simulink model "acac_robust_optimized_r2024a"  (R2024a)
settings: Solver=daessc  StartTime=0  StopTime=0.4  MaxStep=1e-6  RelTol=1e-4
model workspace (MAT data in the model file):
  Fout_Hz = 30
libraries: fl_lib x40, nesl_utility x27, ee_lib x11
(part 1 of 2)
settings Model: Creator=chidan  LastModifiedBy=chidan

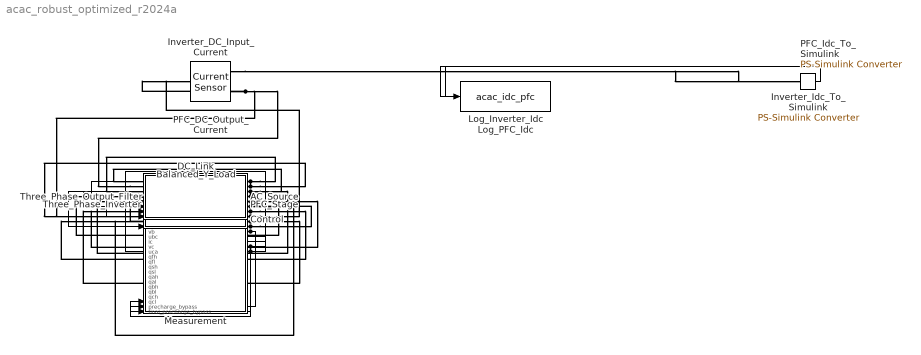
== system acac_robust_optimized_r2024a ==
  AC_Source : Subsystem
  Balanced_Y_Load : Subsystem
  Control : Subsystem
  DC_Link : Subsystem
  Inverter_DC_Input_Current : fl_lib/Electrical/Electrical Sensors/Current Sensor
  Inverter_Idc_To_Simulink : nesl_utility/PS-Simulink Converter  PhysicalDomain=network_engine_domain  SubClassName=ps_output  LeftPortType=input  RightPortType=output  PseudoPeriodic=off  Frequencies=[]  VectorFormat=inherit  Unit=A  AffineConversion=off
  Log_Inverter_Idc : ToWorkspace  VariableName=acac_idc_inverter  SaveFormat=Timeseries  SampleTime=-1
  Log_PFC_Idc : ToWorkspace  VariableName=acac_idc_pfc  SaveFormat=Timeseries  SampleTime=-1
  Measurement : Subsystem
  PFC_DC_Output_Current : fl_lib/Electrical/Electrical Sensors/Current Sensor
  PFC_Idc_To_Simulink : nesl_utility/PS-Simulink Converter  PhysicalDomain=network_engine_domain  SubClassName=ps_output  LeftPortType=input  RightPortType=output  PseudoPeriodic=off  Frequencies=[]  VectorFormat=inherit  Unit=A  AffineConversion=off
  PFC_Stage : Subsystem
  Three_Phase_Inverter : Subsystem
  Three_Phase_Output_Filter : Subsystem
  wires:
  Control/1(QFH) -> PFC_Stage/1(Gate_QFH), Measurement/15(qfh)
  Control/2(QFL) -> PFC_Stage/2(Gate_QFL), Measurement/16(qfl)
  Control/3(QSH) -> PFC_Stage/3(Gate_QSH), Measurement/17(qsh)
  Control/4(QSL) -> PFC_Stage/4(Gate_QSL), Measurement/18(qsl)
  Control/5(QAH) -> Three_Phase_Inverter/1(Gate_AH), Measurement/19(qah)
  Control/6(QAL) -> Three_Phase_Inverter/2(Gate_AL), Measurement/20(qal)
  Control/7(QBH) -> Three_Phase_Inverter/3(Gate_BH), Measurement/21(qbh)
  Control/8(QBL) -> Three_Phase_Inverter/4(Gate_BL), Measurement/22(qbl)
  Control/9(QCH) -> Three_Phase_Inverter/5(Gate_CH), Measurement/23(qch)
  Control/10(QCL) -> Three_Phase_Inverter/6(Gate_CL), Measurement/24(qcl)
  PFC_Stage/1(vin) -> Control/1(vin), Measurement/1(vin)
  PFC_Stage/2(iin) -> Control/2(iin), Measurement/2(iin)
  PFC_Stage/3(vdc) -> Control/3(vdc), Measurement/3(vdc)
  Balanced_Y_Load/2(Va) -> Control/4(va), Measurement/7(va)
  Control/11(PFC_Duty) -> Measurement/4(pfc_duty)
  Control/12(Inverter_Modulation) -> Measurement/5(inverter_modulation)
  Balanced_Y_Load/1(Ia) -> Measurement/6(ia)
  Balanced_Y_Load/3(Uab) -> Measurement/8(uab)
  Balanced_Y_Load/4(Ib) -> Measurement/9(ib)
  Balanced_Y_Load/5(Vb) -> Measurement/10(vb), Control/5(Sense_vb)
  Balanced_Y_Load/6(Ubc) -> Measurement/11(ubc)
  Balanced_Y_Load/7(Ic) -> Measurement/12(ic)
  Balanced_Y_Load/8(Vc) -> Measurement/13(vc), Control/6(Sense_vc)
  Balanced_Y_Load/9(Uca) -> Measurement/14(uca)
  Control/13(Precharge_Bypass) -> PFC_Stage/5(Gate_Precharge_Bypass), Measurement/25(precharge_bypass)
  Control/14(Final_Precharge_Bypass) -> PFC_Stage/6(Gate_Final_Precharge_Bypass), Measurement/26(final_precharge_bypass)
  Inverter_Idc_To_Simulink/1 -> Log_Inverter_Idc/1
  PFC_Idc_To_Simulink/1 -> Log_PFC_Idc/1
  connections:
  AC_Source/RConn1 -- PFC_Stage/LConn1
  AC_Source/RConn2 -- PFC_Stage/LConn2
  DC_Link/LConn2 -- PFC_Stage/RConn2 -- Three_Phase_Inverter/LConn2
  Three_Phase_Inverter/RConn1 -- Three_Phase_Output_Filter/LConn1
  Three_Phase_Inverter/RConn2 -- Three_Phase_Output_Filter/LConn2
  Three_Phase_Inverter/RConn3 -- Three_Phase_Output_Filter/LConn3
  Three_Phase_Output_Filter/RConn1 -- Balanced_Y_Load/LConn1
  Three_Phase_Output_Filter/RConn2 -- Balanced_Y_Load/LConn2
  Three_Phase_Output_Filter/RConn3 -- Balanced_Y_Load/LConn3
  Three_Phase_Output_Filter/RConn4 -- Balanced_Y_Load/LConn4
  Inverter_DC_Input_Current/RConn2 -- Three_Phase_Inverter/LConn1
  Inverter_DC_Input_Current/RConn1 -- Inverter_Idc_To_Simulink/LConn1
  PFC_Stage/RConn1 -- PFC_DC_Output_Current/LConn1
  DC_Link/LConn1 -- PFC_DC_Output_Current/RConn2 -- Inverter_DC_Input_Current/LConn1
  PFC_DC_Output_Current/RConn1 -- PFC_Idc_To_Simulink/LConn1

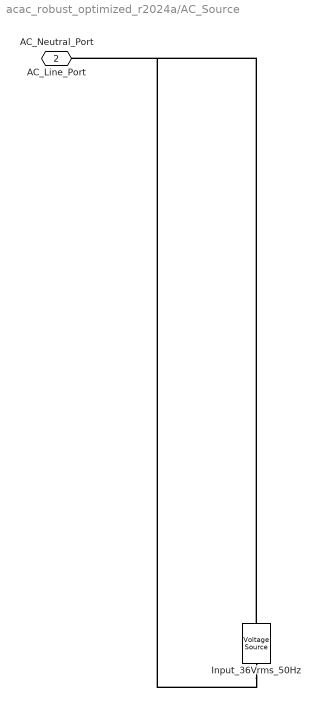
== system acac_robust_optimized_r2024a/AC_Source ==
  Input_36Vrms_50Hz : ee_lib/Sources/Voltage Source  dc_voltage=0 V  ac_voltage=36*sqrt(2) V  ac_shift=0 rad  ac_frequency=50 Hz  noise_mode=ee.enum.sources.noise.Disabled  PSD=0 V^2/Hz  sample_time=1e-3 s  repeatability=ee.enum.sources.repeatability.NotRepeatable  user_seed=0  auto_seed=3499211588  i_specify=off  i_priority=None  i=0 A  i_nominal_specify=off  i_nominal_value=1  i_nominal_unit=A  v_specify=off  v_priority=None  v=0 V  v_nominal_specify=off  v_nominal_value=1  v_nominal_unit=V
  AC_Line_Port : PMIOPort  Side=Right
  AC_Neutral_Port : PMIOPort  Port=2  Side=Right
  connections:
  Input_36Vrms_50Hz/LConn1 -- AC_Line_Port/RConn1
  Input_36Vrms_50Hz/RConn1 -- AC_Neutral_Port/RConn1

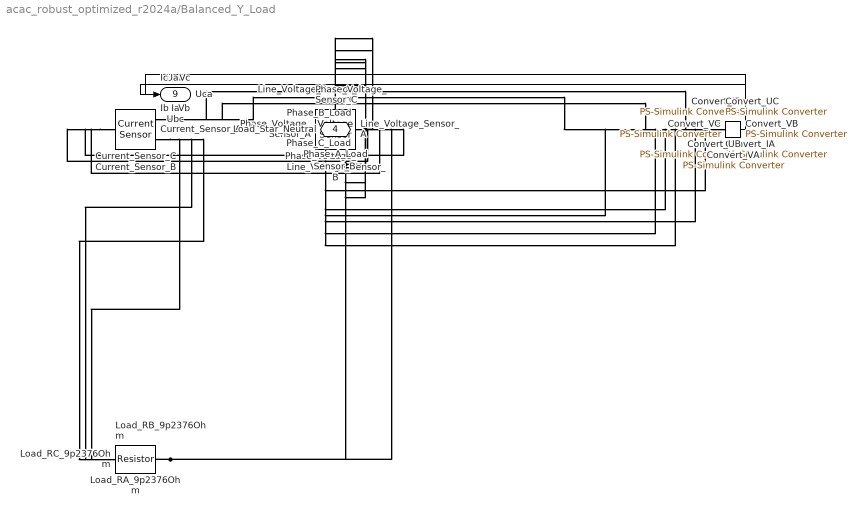
== system acac_robust_optimized_r2024a/Balanced_Y_Load ==
  Convert_IA : nesl_utility/PS-Simulink Converter  PhysicalDomain=network_engine_domain  SubClassName=ps_output  LeftPortType=input  RightPortType=output  PseudoPeriodic=off  Frequencies=[]  VectorFormat=inherit  Unit=inherit  AffineConversion=off
  Convert_IB : nesl_utility/PS-Simulink Converter  PhysicalDomain=network_engine_domain  SubClassName=ps_output  LeftPortType=input  RightPortType=output  PseudoPeriodic=off  Frequencies=[]  VectorFormat=inherit  Unit=inherit  AffineConversion=off
  Convert_IC : nesl_utility/PS-Simulink Converter  PhysicalDomain=network_engine_domain  SubClassName=ps_output  LeftPortType=input  RightPortType=output  PseudoPeriodic=off  Frequencies=[]  VectorFormat=inherit  Unit=inherit  AffineConversion=off
  Convert_UA : nesl_utility/PS-Simulink Converter  PhysicalDomain=network_engine_domain  SubClassName=ps_output  LeftPortType=input  RightPortType=output  PseudoPeriodic=off  Frequencies=[]  VectorFormat=inherit  Unit=inherit  AffineConversion=off
  Convert_UB : nesl_utility/PS-Simulink Converter  PhysicalDomain=network_engine_domain  SubClassName=ps_output  LeftPortType=input  RightPortType=output  PseudoPeriodic=off  Frequencies=[]  VectorFormat=inherit  Unit=inherit  AffineConversion=off
  Convert_UC : nesl_utility/PS-Simulink Converter  PhysicalDomain=network_engine_domain  SubClassName=ps_output  LeftPortType=input  RightPortType=output  PseudoPeriodic=off  Frequencies=[]  VectorFormat=inherit  Unit=inherit  AffineConversion=off
  Convert_VA : nesl_utility/PS-Simulink Converter  PhysicalDomain=network_engine_domain  SubClassName=ps_output  LeftPortType=input  RightPortType=output  PseudoPeriodic=off  Frequencies=[]  VectorFormat=inherit  Unit=inherit  AffineConversion=off
  Convert_VB : nesl_utility/PS-Simulink Converter  PhysicalDomain=network_engine_domain  SubClassName=ps_output  LeftPortType=input  RightPortType=output  PseudoPeriodic=off  Frequencies=[]  VectorFormat=inherit  Unit=inherit  AffineConversion=off
  Convert_VC : nesl_utility/PS-Simulink Converter  PhysicalDomain=network_engine_domain  SubClassName=ps_output  LeftPortType=input  RightPortType=output  PseudoPeriodic=off  Frequencies=[]  VectorFormat=inherit  Unit=inherit  AffineConversion=off
  Current_Sensor_A : fl_lib/Electrical/Electrical Sensors/Current Sensor
  Current_Sensor_B : fl_lib/Electrical/Electrical Sensors/Current Sensor
  Current_Sensor_C : fl_lib/Electrical/Electrical Sensors/Current Sensor
  Line_Voltage_Sensor_A : fl_lib/Electrical/Electrical Sensors/Voltage Sensor
  Line_Voltage_Sensor_B : fl_lib/Electrical/Electrical Sensors/Voltage Sensor
  Line_Voltage_Sensor_C : fl_lib/Electrical/Electrical Sensors/Voltage Sensor
  Load_RA_9p2376Ohm : fl_lib/Electrical/Electrical Elements/Resistor  R=9.237604307 Ohm  i_specify=off  i_priority=None  i=0 A  i_nominal_specify=off  i_nominal_value=1  i_nominal_unit=A  v_specify=off  v_priority=None  v=0 V  v_nominal_specify=off  v_nominal_value=1  v_nominal_unit=V
  Load_RB_9p2376Ohm : fl_lib/Electrical/Electrical Elements/Resistor  R=9.237604307 Ohm  i_specify=off  i_priority=None  i=0 A  i_nominal_specify=off  i_nominal_value=1  i_nominal_unit=A  v_specify=off  v_priority=None  v=0 V  v_nominal_specify=off  v_nominal_value=1  v_nominal_unit=V
  Load_RC_9p2376Ohm : fl_lib/Electrical/Electrical Elements/Resistor  R=9.237604307 Ohm  i_specify=off  i_priority=None  i=0 A  i_nominal_specify=off  i_nominal_value=1  i_nominal_unit=A  v_specify=off  v_priority=None  v=0 V  v_nominal_specify=off  v_nominal_value=1  v_nominal_unit=V
  Phase_Voltage_Sensor_A : fl_lib/Electrical/Electrical Sensors/Voltage Sensor
  Phase_Voltage_Sensor_B : fl_lib/Electrical/Electrical Sensors/Voltage Sensor
  Phase_Voltage_Sensor_C : fl_lib/Electrical/Electrical Sensors/Voltage Sensor
  Phase_A_Load : PMIOPort  Side=Left
  Phase_B_Load : PMIOPort  Port=2  Side=Left
  Phase_C_Load : PMIOPort  Port=3  Side=Left
  Load_Star_Neutral : PMIOPort  Port=4  Side=Left
  Ia : Outport
  Va : Outport  Port=2
  Uab : Outport  Port=3
  Ib : Outport  Port=4
  Vb : Outport  Port=5
  Ubc : Outport  Port=6
  Ic : Outport  Port=7
  Vc : Outport  Port=8
  Uca : Outport  Port=9
  wires:
  Convert_IA/1 -> Ia/1
  Convert_VA/1 -> Va/1
  Convert_IB/1 -> Ib/1
  Convert_VB/1 -> Vb/1
  Convert_IC/1 -> Ic/1
  Convert_VC/1 -> Vc/1
  Convert_UA/1 -> Uab/1
  Convert_UB/1 -> Ubc/1
  Convert_UC/1 -> Uca/1
  connections:
  Current_Sensor_A/LConn1 -- Phase_A_Load/RConn1 -- Phase_Voltage_Sensor_A/LConn1 -- Line_Voltage_Sensor_A/LConn1 -- Line_Voltage_Sensor_C/RConn2
  Current_Sensor_A/RConn2 -- Load_RA_9p2376Ohm/LConn1
  Phase_Voltage_Sensor_A/RConn2 -- Load_Star_Neutral/RConn1 -- Load_RA_9p2376Ohm/RConn1 -- Phase_Voltage_Sensor_B/RConn2 -- Phase_Voltage_Sensor_C/RConn2 -- Load_RB_9p2376Ohm/RConn1 -- Load_RC_9p2376Ohm/RConn1
  Current_Sensor_B/LConn1 -- Phase_B_Load/RConn1 -- Phase_Voltage_Sensor_B/LConn1 -- Line_Voltage_Sensor_A/RConn2 -- Line_Voltage_Sensor_B/LConn1
  Current_Sensor_B/RConn2 -- Load_RB_9p2376Ohm/LConn1
  Current_Sensor_C/LConn1 -- Phase_C_Load/RConn1 -- Phase_Voltage_Sensor_C/LConn1 -- Line_Voltage_Sensor_B/RConn2 -- Line_Voltage_Sensor_C/LConn1
  Current_Sensor_C/RConn2 -- Load_RC_9p2376Ohm/LConn1
  Current_Sensor_A/RConn1 -- Convert_IA/LConn1
  Current_Sensor_B/RConn1 -- Convert_IB/LConn1
  Current_Sensor_C/RConn1 -- Convert_IC/LConn1
  Phase_Voltage_Sensor_A/RConn1 -- Convert_VA/LConn1
  Phase_Voltage_Sensor_B/RConn1 -- Convert_VB/LConn1
  Phase_Voltage_Sensor_C/RConn1 -- Convert_VC/LConn1
  Line_Voltage_Sensor_A/RConn1 -- Convert_UA/LConn1
  Line_Voltage_Sensor_B/RConn1 -- Convert_UB/LConn1
  Line_Voltage_Sensor_C/RConn1 -- Convert_UC/LConn1

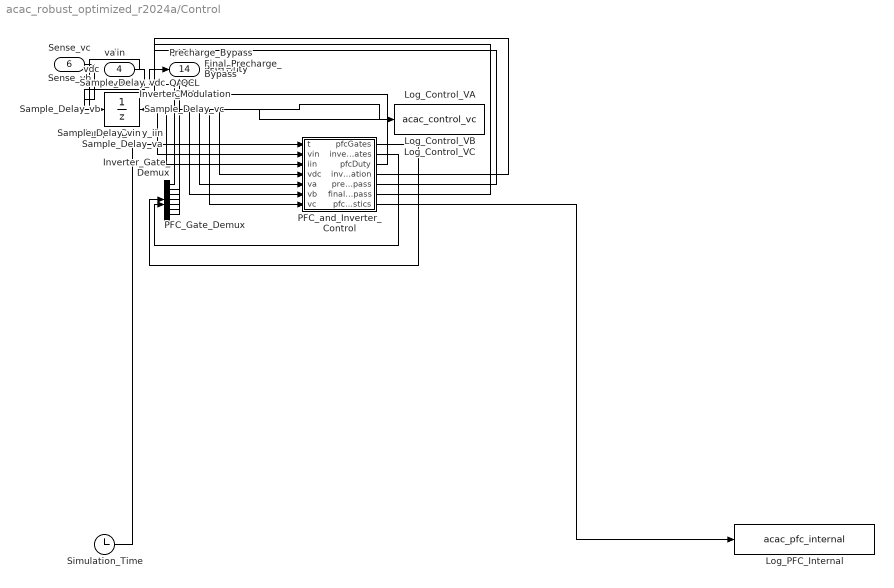
== system acac_robust_optimized_r2024a/Control ==
  vin : Inport
  iin : Inport  Port=2
  vdc : Inport  Port=3
  va : Inport  Port=4
  Sense_vb : Inport  Port=5
  Sense_vc : Inport  Port=6
  Inverter_Gate_Demux : Demux  Outputs=6
  Log_Control_VA : ToWorkspace  VariableName=acac_control_va  SaveFormat=Timeseries  SampleTime=-1
  Log_Control_VB : ToWorkspace  VariableName=acac_control_vb  SaveFormat=Timeseries  SampleTime=-1
  Log_Control_VC : ToWorkspace  VariableName=acac_control_vc  SaveFormat=Timeseries  SampleTime=-1
  Log_PFC_Internal : ToWorkspace  VariableName=acac_pfc_internal  SaveFormat=Timeseries  SampleTime=-1
      settings: Decimation=10
  PFC_Gate_Demux : Demux
  PFC_and_Inverter_Control : MATLAB Function  TreatAsAtomicUnit=on  SystemSampleTime=1e-6
  Sample_Delay_iin : UnitDelay  SampleTime=1e-6  HasFrameUpgradeWarning=on
  Sample_Delay_va : UnitDelay  SampleTime=1e-6  HasFrameUpgradeWarning=on
  Sample_Delay_vb : UnitDelay  SampleTime=1e-6  HasFrameUpgradeWarning=on
  Sample_Delay_vc : UnitDelay  SampleTime=1e-6  HasFrameUpgradeWarning=on
  Sample_Delay_vdc : UnitDelay  SampleTime=1e-6  HasFrameUpgradeWarning=on
  Sample_Delay_vin : UnitDelay  SampleTime=1e-6  HasFrameUpgradeWarning=on
  Simulation_Time : Clock
  QFH : Outport
  QFL : Outport  Port=2
  QSH : Outport  Port=3
  QSL : Outport  Port=4
  QAH : Outport  Port=5
  QAL : Outport  Port=6
  QBH : Outport  Port=7
  QBL : Outport  Port=8
  QCH : Outport  Port=9
  QCL : Outport  Port=10
  PFC_Duty : Outport  Port=11
  Inverter_Modulation : Outport  Port=12
  Precharge_Bypass : Outport  Port=13
  Final_Precharge_Bypass : Outport  Port=14
  wires:
  Simulation_Time/1 -> PFC_and_Inverter_Control/1(t)
  PFC_and_Inverter_Control/1(pfcGates) -> PFC_Gate_Demux/1
  PFC_and_Inverter_Control/2(inverterGates) -> Inverter_Gate_Demux/1
  PFC_and_Inverter_Control/3(pfcDuty) -> PFC_Duty/1
  PFC_and_Inverter_Control/4(inverterModulation) -> Inverter_Modulation/1
  PFC_Gate_Demux/1 -> QFH/1
  PFC_Gate_Demux/2 -> QFL/1
  PFC_Gate_Demux/3 -> QSH/1
  PFC_Gate_Demux/4 -> QSL/1
  Inverter_Gate_Demux/1 -> QAH/1
  Inverter_Gate_Demux/2 -> QAL/1
  Inverter_Gate_Demux/3 -> QBH/1
  Inverter_Gate_Demux/4 -> QBL/1
  Inverter_Gate_Demux/5 -> QCH/1
  Inverter_Gate_Demux/6 -> QCL/1
  vin/1 -> Sample_Delay_vin/1
  Sample_Delay_vin/1 -> PFC_and_Inverter_Control/2(vin)
  iin/1 -> Sample_Delay_iin/1
  Sample_Delay_iin/1 -> PFC_and_Inverter_Control/3(iin)
  vdc/1 -> Sample_Delay_vdc/1
  Sample_Delay_vdc/1 -> PFC_and_Inverter_Control/4(vdc)
  va/1 -> Sample_Delay_va/1
  Sample_Delay_va/1 -> PFC_and_Inverter_Control/5(va), Log_Control_VA/1
  PFC_and_Inverter_Control/5(prechargeBypass) -> Precharge_Bypass/1
  PFC_and_Inverter_Control/6(finalPrechargeBypass) -> Final_Precharge_Bypass/1
  Sense_vb/1 -> Sample_Delay_vb/1
  Sample_Delay_vb/1 -> PFC_and_Inverter_Control/6(vb), Log_Control_VB/1
  Sense_vc/1 -> Sample_Delay_vc/1
  Sample_Delay_vc/1 -> PFC_and_Inverter_Control/7(vc), Log_Control_VC/1
  PFC_and_Inverter_Control/7(pfcDiagnostics) -> Log_PFC_Internal/1

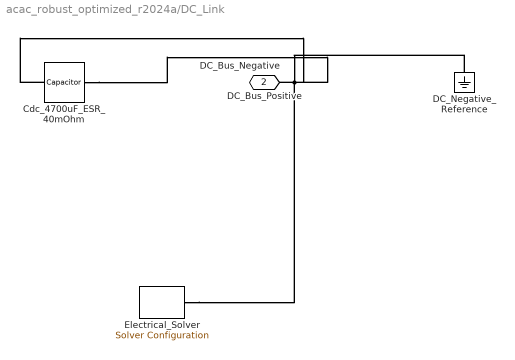
== system acac_robust_optimized_r2024a/DC_Link ==
  Cdc_4700uF_ESR_40mOhm : fl_lib/Electrical/Electrical Elements/Capacitor  c=4.7e-3 F  r=0.04 Ohm  g=0 1/Ohm  i_specify=off  i_priority=None  i=0 A  i_nominal_specify=off  i_nominal_value=1  i_nominal_unit=A  v_specify=off  v_priority=None  v=0 V  v_nominal_specify=off  v_nominal_value=1  v_nominal_unit=V  vc_specify=off  vc_priority=High  vc=0 V  vc_nominal_specify=off  vc_nominal_value=1  vc_nominal_unit=V
  DC_Negative_Reference : fl_lib/Electrical/Electrical Elements/Electrical Reference
  Electrical_Solver : nesl_utility/Solver Configuration  PhysicalDomain=network_engine_domain  SubClassName=solver  LeftPortType=input  RightPortType=generic  Tones=[]  Harmonics=[]  SimulateNoise=off  Profile=off  UseLocalSampling=off  EnableSwitchedLinearOptims=on  FrequencyDomain=off  UseCCode=off  RelTol=0.001  AbsTol=0.001  MinStep=1e-09  ToWorkspace=off  RevertToSquareIcSolve=off  NumHomotopyIterations=100  PhasorMode=off  PhasorModeNumHarmonics=1  ConsistencySolver=NEWTON_XTOL_AFTER_FTOL  IndexReductionMethod=DerivativeReplacement  DoDC=off  ResidualTolerance=1e-09  ConsistencyTolSource=GLOBAL  ConsistencyAbsTol=0.001  ConsistencyRelTol=0.001  ConsistencyTolFactor=0.001  UseLocalSolver=off  LocalSolverChoice=NE_BACKWARD_EULER_ADVANCER  ResolveIndetEquations=on  FunctionEvalNumThread=1  LocalSolverSampleTime=0.001  DoFixedCost=off  MaxNonlinIter=3  MaxModeIter=2  ComputeImpulses=off  ImpulseIterations=2  LinearAlgebra=auto  LinearAlgebraNumThread=0  EquationFormulation=NE_TIME_EF  DelaysMemoryBudget=1024  AutomaticFiltering=on  FilteringTimeConstant=0.001  PartitionStorageMethod=AS_NEEDED  PartitionMemoryBudget=1024  PartitionMethod=ROBUST  MultibodyUseLocalSolver=off  MultibodyLocalSolverChoice=ODE1  MultibodyLocalSolverSampleTime=0.001
  DC_Bus_Positive : PMIOPort  Side=Left
  DC_Bus_Negative : PMIOPort  Port=2  Side=Left
  connections:
  Cdc_4700uF_ESR_40mOhm/LConn1 -- DC_Bus_Positive/RConn1
  Cdc_4700uF_ESR_40mOhm/RConn1 -- DC_Negative_Reference/LConn1 -- DC_Bus_Negative/RConn1 -- Electrical_Solver/RConn1

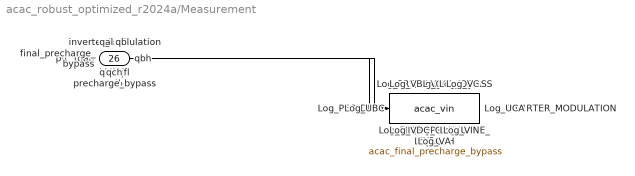
== system acac_robust_optimized_r2024a/Measurement ==
  vin : Inport
  iin : Inport  Port=2
  vdc : Inport  Port=3
  pfc_duty : Inport  Port=4
  inverter_modulation : Inport  Port=5
  ia : Inport  Port=6
  va : Inport  Port=7
  uab : Inport  Port=8
  ib : Inport  Port=9
  vb : Inport  Port=10
  ubc : Inport  Port=11
  ic : Inport  Port=12
  vc : Inport  Port=13
  uca : Inport  Port=14
  qfh : Inport  Port=15
  qfl : Inport  Port=16
  qsh : Inport  Port=17
  qsl : Inport  Port=18
  qah : Inport  Port=19
  qal : Inport  Port=20
  qbh : Inport  Port=21
  qbl : Inport  Port=22
  qch : Inport  Port=23
  qcl : Inport  Port=24
  precharge_bypass : Inport  Port=25
  final_precharge_bypass : Inport  Port=26
  Log_FINAL_PRECHARGE_BYPASS : ToWorkspace  VariableName=acac_final_precharge_bypass  SaveFormat=Timeseries  SampleTime=-1
  Log_IA : ToWorkspace  VariableName=acac_ia  SaveFormat=Timeseries  SampleTime=-1
  Log_IB : ToWorkspace  VariableName=acac_ib  SaveFormat=Timeseries  SampleTime=-1
  Log_IC : ToWorkspace  VariableName=acac_ic  SaveFormat=Timeseries  SampleTime=-1
  Log_IIN : ToWorkspace  VariableName=acac_iin  SaveFormat=Timeseries  SampleTime=-1
  Log_INVERTER_MODULATION : ToWorkspace  VariableName=acac_inverter_modulation  SaveFormat=Timeseries  SampleTime=-1
  Log_PFC_DUTY : ToWorkspace  VariableName=acac_pfc_duty  SaveFormat=Timeseries  SampleTime=-1
  Log_PRECHARGE_BYPASS : ToWorkspace  VariableName=acac_precharge_bypass  SaveFormat=Timeseries  SampleTime=-1
  Log_QAH : ToWorkspace  VariableName=acac_qah  SaveFormat=Timeseries  SampleTime=-1
  Log_QAL : ToWorkspace  VariableName=acac_qal  SaveFormat=Timeseries  SampleTime=-1
  Log_QBH : ToWorkspace  VariableName=acac_qbh  SaveFormat=Timeseries  SampleTime=-1
  Log_QBL : ToWorkspace  VariableName=acac_qbl  SaveFormat=Timeseries  SampleTime=-1
  Log_QCH : ToWorkspace  VariableName=acac_qch  SaveFormat=Timeseries  SampleTime=-1
  Log_QCL : ToWorkspace  VariableName=acac_qcl  SaveFormat=Timeseries  SampleTime=-1
  Log_QFH : ToWorkspace  VariableName=acac_qfh  SaveFormat=Timeseries  SampleTime=-1
  Log_QFL : ToWorkspace  VariableName=acac_qfl  SaveFormat=Timeseries  SampleTime=-1
  Log_QSH : ToWorkspace  VariableName=acac_qsh  SaveFormat=Timeseries  SampleTime=-1
  Log_QSL : ToWorkspace  VariableName=acac_qsl  SaveFormat=Timeseries  SampleTime=-1
  Log_UAB : ToWorkspace  VariableName=acac_uab  SaveFormat=Timeseries  SampleTime=-1
  Log_UBC : ToWorkspace  VariableName=acac_ubc  SaveFormat=Timeseries  SampleTime=-1
  Log_UCA : ToWorkspace  VariableName=acac_uca  SaveFormat=Timeseries  SampleTime=-1
  Log_VA : ToWorkspace  VariableName=acac_va  SaveFormat=Timeseries  SampleTime=-1
  Log_VB : ToWorkspace  VariableName=acac_vb  SaveFormat=Timeseries  SampleTime=-1
  Log_VC : ToWorkspace  VariableName=acac_vc  SaveFormat=Timeseries  SampleTime=-1
  Log_VDC : ToWorkspace  VariableName=acac_vdc  SaveFormat=Timeseries  SampleTime=-1
  Log_VIN : ToWorkspace  VariableName=acac_vin  SaveFormat=Timeseries  SampleTime=-1
  wires:
  vin/1 -> Log_VIN/1
  iin/1 -> Log_IIN/1
  vdc/1 -> Log_VDC/1
  pfc_duty/1 -> Log_PFC_DUTY/1
  inverter_modulation/1 -> Log_INVERTER_MODULATION/1
  ia/1 -> Log_IA/1
  va/1 -> Log_VA/1
  uab/1 -> Log_UAB/1
  ib/1 -> Log_IB/1
  vb/1 -> Log_VB/1
  ubc/1 -> Log_UBC/1
  ic/1 -> Log_IC/1
  vc/1 -> Log_VC/1
  uca/1 -> Log_UCA/1
  qfh/1 -> Log_QFH/1
  qfl/1 -> Log_QFL/1
  qsh/1 -> Log_QSH/1
  qsl/1 -> Log_QSL/1
  qah/1 -> Log_QAH/1
  qal/1 -> Log_QAL/1
  qbh/1 -> Log_QBH/1
  qbl/1 -> Log_QBL/1
  qch/1 -> Log_QCH/1
  qcl/1 -> Log_QCL/1
  precharge_bypass/1 -> Log_PRECHARGE_BYPASS/1
  final_precharge_bypass/1 -> Log_FINAL_PRECHARGE_BYPASS/1

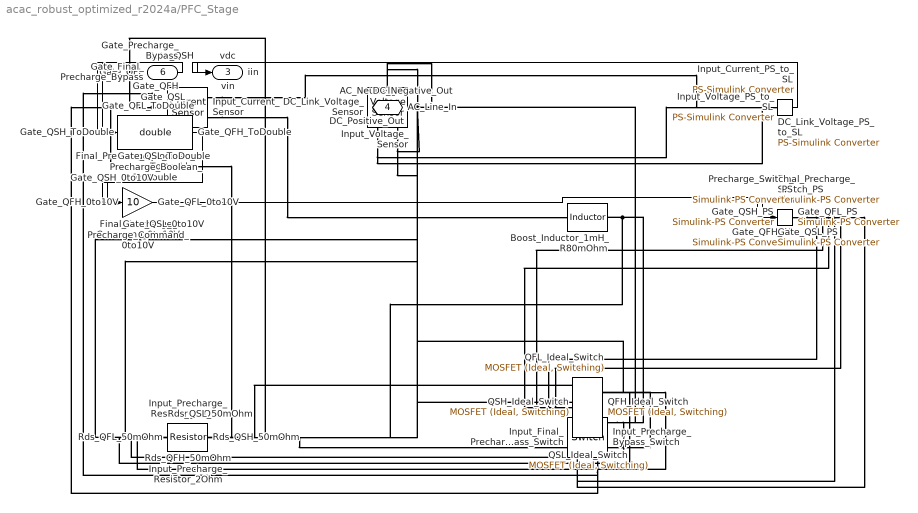
== system acac_robust_optimized_r2024a/PFC_Stage ==
  Gate_QFH : Inport
  Gate_QFL : Inport  Port=2
  Gate_QSH : Inport  Port=3
  Gate_QSL : Inport  Port=4
  Gate_Precharge_Bypass : Inport  Port=5
  Gate_Final_Precharge_Bypass : Inport  Port=6
  Boost_Inductor_1mH_R80mOhm : fl_lib/Electrical/Electrical Elements/Inductor  l=1e-3 H  r=0.08 Ohm  g=1e-9 1/Ohm  i_specify=off  i_priority=None  i=0 A  i_nominal_specify=off  i_nominal_value=1  i_nominal_unit=A  v_specify=off  v_priority=None  v=0 V  v_nominal_specify=off  v_nominal_value=1  v_nominal_unit=V  i_L_specify=off  i_L_priority=High  i_L=0 A  i_L_nominal_specify=off  i_L_nominal_value=1  i_L_nominal_unit=A
  DC_Link_Voltage_PS_to_SL : nesl_utility/PS-Simulink Converter  PhysicalDomain=network_engine_domain  SubClassName=ps_output  LeftPortType=input  RightPortType=output  PseudoPeriodic=off  Frequencies=[]  VectorFormat=inherit  Unit=inherit  AffineConversion=off
  DC_Link_Voltage_Sensor : fl_lib/Electrical/Electrical Sensors/Voltage Sensor
  Final_Precharge_Boolean_ToDouble : DataTypeConversion  OutDataTypeStr=double  SaturateOnIntegerOverflow=off  RndMeth=Floor
  Final_Precharge_Command_0to10V : Gain  Gain=10
  Final_Precharge_Switch_PS : nesl_utility/Simulink-PS Converter  PhysicalDomain=network_engine_domain  SubClassName=ps_input  LeftPortType=input  RightPortType=output  PseudoPeriodic=off  Frequencies=[]  NoiseDistribution=none  NoiseParameters=[]  Unit=1  AffineConversion=off  FilteringAndDerivatives=provide  SimscapeFilterOrder=1  InputFilterTimeConstant=0.001  UdotUserProvided=0
  Gate_QFH_0to10V : Gain  Gain=10
  Gate_QFH_PS : nesl_utility/Simulink-PS Converter  PhysicalDomain=network_engine_domain  SubClassName=ps_input  LeftPortType=input  RightPortType=output  PseudoPeriodic=off  Frequencies=[]  NoiseDistribution=none  NoiseParameters=[]  Unit=1  AffineConversion=off  FilteringAndDerivatives=provide  SimscapeFilterOrder=1  InputFilterTimeConstant=0.001  UdotUserProvided=0
  Gate_QFH_ToDouble : DataTypeConversion  OutDataTypeStr=double  SaturateOnIntegerOverflow=off  RndMeth=Floor
  Gate_QFL_0to10V : Gain  Gain=10
  Gate_QFL_PS : nesl_utility/Simulink-PS Converter  PhysicalDomain=network_engine_domain  SubClassName=ps_input  LeftPortType=input  RightPortType=output  PseudoPeriodic=off  Frequencies=[]  NoiseDistribution=none  NoiseParameters=[]  Unit=1  AffineConversion=off  FilteringAndDerivatives=provide  SimscapeFilterOrder=1  InputFilterTimeConstant=0.001  UdotUserProvided=0
  Gate_QFL_ToDouble : DataTypeConversion  OutDataTypeStr=double  SaturateOnIntegerOverflow=off  RndMeth=Floor
  Gate_QSH_0to10V : Gain  Gain=10
  Gate_QSH_PS : nesl_utility/Simulink-PS Converter  PhysicalDomain=network_engine_domain  SubClassName=ps_input  LeftPortType=input  RightPortType=output  PseudoPeriodic=off  Frequencies=[]  NoiseDistribution=none  NoiseParameters=[]  Unit=1  AffineConversion=off  FilteringAndDerivatives=provide  SimscapeFilterOrder=1  InputFilterTimeConstant=0.001  UdotUserProvided=0
  Gate_QSH_ToDouble : DataTypeConversion  OutDataTypeStr=double  SaturateOnIntegerOverflow=off  RndMeth=Floor
  Gate_QSL_0to10V : Gain  Gain=10
  Gate_QSL_PS : nesl_utility/Simulink-PS Converter  PhysicalDomain=network_engine_domain  SubClassName=ps_input  LeftPortType=input  RightPortType=output  PseudoPeriodic=off  Frequencies=[]  NoiseDistribution=none  NoiseParameters=[]  Unit=1  AffineConversion=off  FilteringAndDerivatives=provide  SimscapeFilterOrder=1  InputFilterTimeConstant=0.001  UdotUserProvided=0
  Gate_QSL_ToDouble : DataTypeConversion  OutDataTypeStr=double  SaturateOnIntegerOverflow=off  RndMeth=Floor
  Input_Current_PS_to_SL : nesl_utility/PS-Simulink Converter  PhysicalDomain=network_engine_domain  SubClassName=ps_output  LeftPortType=input  RightPortType=output  PseudoPeriodic=off  Frequencies=[]  VectorFormat=inherit  Unit=inherit  AffineConversion=off
  Input_Current_Sensor : fl_lib/Electrical/Electrical Sensors/Current Sensor
  Input_Final_Precharge_Bypass_Switch : fl_lib/Electrical/Electrical Elements/Switch  R_closed=0.01 Ohm  G_open=1e-8 1/Ohm  Threshold=0.5  i_specify=off  i_priority=None  i=0 A  i_nominal_specify=off  i_nominal_value=1  i_nominal_unit=A  v_specify=off  v_priority=None  v=0 V  v_nominal_specify=off  v_nominal_value=1  v_nominal_unit=V
  Input_Precharge_Bypass_Switch : fl_lib/Electrical/Electrical Elements/Switch  R_closed=0.01 Ohm  G_open=1e-8 1/Ohm  Threshold=0.5  i_specify=off  i_priority=None  i=0 A  i_nominal_specify=off  i_nominal_value=1  i_nominal_unit=A  v_specify=off  v_priority=None  v=0 V  v_nominal_specify=off  v_nominal_value=1  v_nominal_unit=V
  Input_Precharge_Resistor_10Ohm : fl_lib/Electrical/Electrical Elements/Resistor  R=10 Ohm  i_specify=off  i_priority=None  i=0 A  i_nominal_specify=off  i_nominal_value=1  i_nominal_unit=A  v_specify=off  v_priority=None  v=0 V  v_nominal_specify=off  v_nominal_value=1  v_nominal_unit=V
  Input_Precharge_Resistor_2Ohm : fl_lib/Electrical/Electrical Elements/Resistor  R=2 Ohm  i_specify=off  i_priority=None  i=0 A  i_nominal_specify=off  i_nominal_value=1  i_nominal_unit=A  v_specify=off  v_priority=None  v=0 V  v_nominal_specify=off  v_nominal_value=1  v_nominal_unit=V
  Input_Voltage_PS_to_SL : nesl_utility/PS-Simulink Converter  PhysicalDomain=network_engine_domain  SubClassName=ps_output  LeftPortType=input  RightPortType=output  PseudoPeriodic=off  Frequencies=[]  VectorFormat=inherit  Unit=inherit  AffineConversion=off
  Input_Voltage_Sensor : fl_lib/Electrical/Electrical Sensors/Voltage Sensor
  Precharge_Boolean_ToDouble : DataTypeConversion  OutDataTypeStr=double  SaturateOnIntegerOverflow=off  RndMeth=Floor
  Precharge_Command_0to10V : Gain  Gain=10
  Precharge_Switch_PS : nesl_utility/Simulink-PS Converter  PhysicalDomain=network_engine_domain  SubClassName=ps_input  LeftPortType=input  RightPortType=output  PseudoPeriodic=off  Frequencies=[]  NoiseDistribution=none  NoiseParameters=[]  Unit=1  AffineConversion=off  FilteringAndDerivatives=provide  SimscapeFilterOrder=1  InputFilterTimeConstant=0.001  UdotUserProvided=0
  QFH_Ideal_Switch : ee_lib/Semiconductors & Converters/MOSFET (Ideal, Switching)  port_option=ee.enum.controlport.ps  Rds=0.01 Ohm  Goff=1e-6 1/Ohm  Vth=2 V  diode_param=ee.enum.semiconductors.protectionDiode.nodynamics  diode_Vf=0.8 V  diode_Ron=0.001 Ohm  diode_Goff=1e-5 1/Ohm  diode_C=50e-9 F  diode_iRM=-235 A  diode_iF=300 A  diode_idot=-50 A/us  diode_trr_param=ee.enum.converters.diodeReverseParam.trr_factor  diode_trr_factor=3  diode_trr=15 us  diode_Qrr=1500 s*uA  ids_specify=off  ids_priority=None  ids=0 A  ids_nominal_specify=off  ids_nominal_value=1  ids_nominal_unit=A  vds_specify=off  vds_priority=None  vds=0 V  vds_nominal_specify=off  vds_nominal_value=1  vds_nominal_unit=V  vgs_specify=off  vgs_priority=None  vgs=0 V  vgs_nominal_specify=off  vgs_nominal_value=1  vgs_nominal_unit=V  thermal_loss_option=ee.enum.converters.thermalLossOption.constantvalues  Von_data=[0, 1.8, 3.2, 6, 10, 16; 0, 2, 5.5, 9.5, 15, 25] V  Tj=[298.15, 448.15] K  Iout_data=[0, 20, 40, 60, 80, 100] A  Eon_data=[0, 55.04, 124.57, 235.53, 362.12; 0, 71.25, 161.25, 304.88, 468.75] * 1e-6 J  Eoff_data=[0, 18, 30, 56.1, 76.5; 0, 22.5, 37.5, 70.13, 95.63] * 1e-6 J  Eon_data_3D=[zeros(2, 5, 3)] J  Eoff_data_3D=[zeros(2, 5, 3)] J  Tj_loss=[298.15, 448.15] K  Iout_data_loss=[0, 10, 20, 30, 40] A  tabulateWithVds=false  Vds_loss=[0, 150, 300] V  Eon_scalar=22.86e-3 J  Eoff_scalar=17.14e-3 J  Voff=300 V  Iout_scalar=600 A  useCurrentFromPreviousCycle=false  useVoltageFromPreviousCycle=false  diodeModelType=ee.enum.converters.diodeModelType.pwl  diodeTableType=ee.enum.diode.tableType.IfMat  diode_ReverseIVType=ee.enum.diode.diodeReverseIV.constant  diode_IfMat=[.07, .12, .19, 1.75, 4.24, 7.32, 11.2; .16, .3, .72, 2.14, 4.02, 6.35, 9.12] A  diode_VfMat=[.9, 1.15, 1.25, 1.5, 1.75, 2.17, 2.6, 2.85; .58, .68, .75, 1.1, 1.38, 1.77, 2.27, 2.7] V  diode_TjVec=[25, 125] degC  diode_VfVec=[.5, .7, .9, 1.3, 1.7, 2.1, 2.5] V  diode_IfVec=[.1, .2, .5, 1, 2, 4, 7, 10] A  diode_IrMat=[1e-06, 2e-06, 5e-06, 1e-05, 2.5e-05, 5e-05, .0001; 2e-06, 5e-06, 1e-05, 4e-05, 8e-05, .0002, .0005] A  diode_VrMat=[10, 100, 200, 250, 300, 325, 350; 10, 70, 160, 220, 270, 300, 320] V  diode_VrVec=[10, 20, 40, 50, 70, 80, 100] V  diode_IrVec=[1e-06, 2e-06, 5e-06, 1e-05, 2e-05, 5e-05, .0001] A  diode_Vr=-600 V  diode_Ls=150 nH  diode_Erec=0.03 J  diode_rec_loss_model=ee.enum.diode.reverseRecoveryModel.fixed  diode_ErecVal=0 J  diode_scaleWithIandV=true  diode_ErecMat=zeros(2, 3) J  diode_TjrecVec=[298.15, 398.15] K  diode_IfrecVec=[.1, 1, 10] A  diode_IrecVal=10 A  diode_VrecVal=10 V  diode_tFilter=1 / 1000 / 100 s  thermal_network_parameterization=ee.enum.thermalNetworkTopology.external  Rth=[.03, .2] K/W  Rth_Cauer=[.03, .1, .2] K/W  Rth_Foster=[.03, .2] K/W  thermal_mass_parameterization=ee.enum.thermalNetwork.timeconstant  thermal_mass=[3, 25] J/K  thermal_mass_Cauer=[3, 10, 25] J/K  thermal_mass_Foster=[33, 50] J/K  thermal_time_constant=[.1, 5] s  thermal_time_constant_Cauer=[.1, 1, 5] s  thermal_time_constant_Foster=[1, 10] s  thermal_mass_initial_temperatures=[25, 25] degC  thermal_mass_initial_temperatures_Cauer=[25, 25, 25] degC  junction_thermal_mass=0.1 J/K  Tvec_initial_Foster=[25, 25, 25, 25] degC  no_thermal_network=0  junction_temperature_specify=off  junction_temperature_priority=None  junction_temperature=25 degC  junction_temperature_nominal_specify=off  junction_temperature_nominal_value=1  junction_temperature_nominal_unit=degC  Qj_specify=off  Qj_priority=None  Qj=0 W  Qj_nominal_specify=off  Qj_nominal_value=1  Qj_nominal_unit=W  accumulatedSwitchingLosses_specify=off  accumulatedSwitchingLosses_priority=None  accumulatedSwitchingLosses=0 J
  QFL_Ideal_Switch : ee_lib/Semiconductors & Converters/MOSFET (Ideal, Switching)  port_option=ee.enum.controlport.ps  Rds=0.01 Ohm  Goff=1e-6 1/Ohm  Vth=2 V  diode_param=ee.enum.semiconductors.protectionDiode.nodynamics  diode_Vf=0.8 V  diode_Ron=0.001 Ohm  diode_Goff=1e-5 1/Ohm  diode_C=50e-9 F  diode_iRM=-235 A  diode_iF=300 A  diode_idot=-50 A/us  diode_trr_param=ee.enum.converters.diodeReverseParam.trr_factor  diode_trr_factor=3  diode_trr=15 us  diode_Qrr=1500 s*uA  ids_specify=off  ids_priority=None  ids=0 A  ids_nominal_specify=off  ids_nominal_value=1  ids_nominal_unit=A  vds_specify=off  vds_priority=None  vds=0 V  vds_nominal_specify=off  vds_nominal_value=1  vds_nominal_unit=V  vgs_specify=off  vgs_priority=None  vgs=0 V  vgs_nominal_specify=off  vgs_nominal_value=1  vgs_nominal_unit=V  thermal_loss_option=ee.enum.converters.thermalLossOption.constantvalues  Von_data=[0, 1.8, 3.2, 6, 10, 16; 0, 2, 5.5, 9.5, 15, 25] V  Tj=[298.15, 448.15] K  Iout_data=[0, 20, 40, 60, 80, 100] A  Eon_data=[0, 55.04, 124.57, 235.53, 362.12; 0, 71.25, 161.25, 304.88, 468.75] * 1e-6 J  Eoff_data=[0, 18, 30, 56.1, 76.5; 0, 22.5, 37.5, 70.13, 95.63] * 1e-6 J  Eon_data_3D=[zeros(2, 5, 3)] J  Eoff_data_3D=[zeros(2, 5, 3)] J  Tj_loss=[298.15, 448.15] K  Iout_data_loss=[0, 10, 20, 30, 40] A  tabulateWithVds=false  Vds_loss=[0, 150, 300] V  Eon_scalar=22.86e-3 J  Eoff_scalar=17.14e-3 J  Voff=300 V  Iout_scalar=600 A  useCurrentFromPreviousCycle=false  useVoltageFromPreviousCycle=false  diodeModelType=ee.enum.converters.diodeModelType.pwl  diodeTableType=ee.enum.diode.tableType.IfMat  diode_ReverseIVType=ee.enum.diode.diodeReverseIV.constant  diode_IfMat=[.07, .12, .19, 1.75, 4.24, 7.32, 11.2; .16, .3, .72, 2.14, 4.02, 6.35, 9.12] A  diode_VfMat=[.9, 1.15, 1.25, 1.5, 1.75, 2.17, 2.6, 2.85; .58, .68, .75, 1.1, 1.38, 1.77, 2.27, 2.7] V  diode_TjVec=[25, 125] degC  diode_VfVec=[.5, .7, .9, 1.3, 1.7, 2.1, 2.5] V  diode_IfVec=[.1, .2, .5, 1, 2, 4, 7, 10] A  diode_IrMat=[1e-06, 2e-06, 5e-06, 1e-05, 2.5e-05, 5e-05, .0001; 2e-06, 5e-06, 1e-05, 4e-05, 8e-05, .0002, .0005] A  diode_VrMat=[10, 100, 200, 250, 300, 325, 350; 10, 70, 160, 220, 270, 300, 320] V  diode_VrVec=[10, 20, 40, 50, 70, 80, 100] V  diode_IrVec=[1e-06, 2e-06, 5e-06, 1e-05, 2e-05, 5e-05, .0001] A  diode_Vr=-600 V  diode_Ls=150 nH  diode_Erec=0.03 J  diode_rec_loss_model=ee.enum.diode.reverseRecoveryModel.fixed  diode_ErecVal=0 J  diode_scaleWithIandV=true  diode_ErecMat=zeros(2, 3) J  diode_TjrecVec=[298.15, 398.15] K  diode_IfrecVec=[.1, 1, 10] A  diode_IrecVal=10 A  diode_VrecVal=10 V  diode_tFilter=1 / 1000 / 100 s  thermal_network_parameterization=ee.enum.thermalNetworkTopology.external  Rth=[.03, .2] K/W  Rth_Cauer=[.03, .1, .2] K/W  Rth_Foster=[.03, .2] K/W  thermal_mass_parameterization=ee.enum.thermalNetwork.timeconstant  thermal_mass=[3, 25] J/K  thermal_mass_Cauer=[3, 10, 25] J/K  thermal_mass_Foster=[33, 50] J/K  thermal_time_constant=[.1, 5] s  thermal_time_constant_Cauer=[.1, 1, 5] s  thermal_time_constant_Foster=[1, 10] s  thermal_mass_initial_temperatures=[25, 25] degC  thermal_mass_initial_temperatures_Cauer=[25, 25, 25] degC  junction_thermal_mass=0.1 J/K  Tvec_initial_Foster=[25, 25, 25, 25] degC  no_thermal_network=0  junction_temperature_specify=off  junction_temperature_priority=None  junction_temperature=25 degC  junction_temperature_nominal_specify=off  junction_temperature_nominal_value=1  junction_temperature_nominal_unit=degC  Qj_specify=off  Qj_priority=None  Qj=0 W  Qj_nominal_specify=off  Qj_nominal_value=1  Qj_nominal_unit=W  accumulatedSwitchingLosses_specify=off  accumulatedSwitchingLosses_priority=None  accumulatedSwitchingLosses=0 J
  QSH_Ideal_Switch : ee_lib/Semiconductors & Converters/MOSFET (Ideal, Switching)  port_option=ee.enum.controlport.ps  Rds=0.01 Ohm  Goff=1e-6 1/Ohm  Vth=2 V  diode_param=ee.enum.semiconductors.protectionDiode.nodynamics  diode_Vf=0.8 V  diode_Ron=0.001 Ohm  diode_Goff=1e-5 1/Ohm  diode_C=50e-9 F  diode_iRM=-235 A  diode_iF=300 A  diode_idot=-50 A/us  diode_trr_param=ee.enum.converters.diodeReverseParam.trr_factor  diode_trr_factor=3  diode_trr=15 us  diode_Qrr=1500 s*uA  ids_specify=off  ids_priority=None  ids=0 A  ids_nominal_specify=off  ids_nominal_value=1  ids_nominal_unit=A  vds_specify=off  vds_priority=None  vds=0 V  vds_nominal_specify=off  vds_nominal_value=1  vds_nominal_unit=V  vgs_specify=off  vgs_priority=None  vgs=0 V  vgs_nominal_specify=off  vgs_nominal_value=1  vgs_nominal_unit=V  thermal_loss_option=ee.enum.converters.thermalLossOption.constantvalues  Von_data=[0, 1.8, 3.2, 6, 10, 16; 0, 2, 5.5, 9.5, 15, 25] V  Tj=[298.15, 448.15] K  Iout_data=[0, 20, 40, 60, 80, 100] A  Eon_data=[0, 55.04, 124.57, 235.53, 362.12; 0, 71.25, 161.25, 304.88, 468.75] * 1e-6 J  Eoff_data=[0, 18, 30, 56.1, 76.5; 0, 22.5, 37.5, 70.13, 95.63] * 1e-6 J  Eon_data_3D=[zeros(2, 5, 3)] J  Eoff_data_3D=[zeros(2, 5, 3)] J  Tj_loss=[298.15, 448.15] K  Iout_data_loss=[0, 10, 20, 30, 40] A  tabulateWithVds=false  Vds_loss=[0, 150, 300] V  Eon_scalar=22.86e-3 J  Eoff_scalar=17.14e-3 J  Voff=300 V  Iout_scalar=600 A  useCurrentFromPreviousCycle=false  useVoltageFromPreviousCycle=false  diodeModelType=ee.enum.converters.diodeModelType.pwl  diodeTableType=ee.enum.diode.tableType.IfMat  diode_ReverseIVType=ee.enum.diode.diodeReverseIV.constant  diode_IfMat=[.07, .12, .19, 1.75, 4.24, 7.32, 11.2; .16, .3, .72, 2.14, 4.02, 6.35, 9.12] A  diode_VfMat=[.9, 1.15, 1.25, 1.5, 1.75, 2.17, 2.6, 2.85; .58, .68, .75, 1.1, 1.38, 1.77, 2.27, 2.7] V  diode_TjVec=[25, 125] degC  diode_VfVec=[.5, .7, .9, 1.3, 1.7, 2.1, 2.5] V  diode_IfVec=[.1, .2, .5, 1, 2, 4, 7, 10] A  diode_IrMat=[1e-06, 2e-06, 5e-06, 1e-05, 2.5e-05, 5e-05, .0001; 2e-06, 5e-06, 1e-05, 4e-05, 8e-05, .0002, .0005] A  diode_VrMat=[10, 100, 200, 250, 300, 325, 350; 10, 70, 160, 220, 270, 300, 320] V  diode_VrVec=[10, 20, 40, 50, 70, 80, 100] V  diode_IrVec=[1e-06, 2e-06, 5e-06, 1e-05, 2e-05, 5e-05, .0001] A  diode_Vr=-600 V  diode_Ls=150 nH  diode_Erec=0.03 J  diode_rec_loss_model=ee.enum.diode.reverseRecoveryModel.fixed  diode_ErecVal=0 J  diode_scaleWithIandV=true  diode_ErecMat=zeros(2, 3) J  diode_TjrecVec=[298.15, 398.15] K  diode_IfrecVec=[.1, 1, 10] A  diode_IrecVal=10 A  diode_VrecVal=10 V  diode_tFilter=1 / 1000 / 100 s  thermal_network_parameterization=ee.enum.thermalNetworkTopology.external  Rth=[.03, .2] K/W  Rth_Cauer=[.03, .1, .2] K/W  Rth_Foster=[.03, .2] K/W  thermal_mass_parameterization=ee.enum.thermalNetwork.timeconstant  thermal_mass=[3, 25] J/K  thermal_mass_Cauer=[3, 10, 25] J/K  thermal_mass_Foster=[33, 50] J/K  thermal_time_constant=[.1, 5] s  thermal_time_constant_Cauer=[.1, 1, 5] s  thermal_time_constant_Foster=[1, 10] s  thermal_mass_initial_temperatures=[25, 25] degC  thermal_mass_initial_temperatures_Cauer=[25, 25, 25] degC  junction_thermal_mass=0.1 J/K  Tvec_initial_Foster=[25, 25, 25, 25] degC  no_thermal_network=0  junction_temperature_specify=off  junction_temperature_priority=None  junction_temperature=25 degC  junction_temperature_nominal_specify=off  junction_temperature_nominal_value=1  junction_temperature_nominal_unit=degC  Qj_specify=off  Qj_priority=None  Qj=0 W  Qj_nominal_specify=off  Qj_nominal_value=1  Qj_nominal_unit=W  accumulatedSwitchingLosses_specify=off  accumulatedSwitchingLosses_priority=None  accumulatedSwitchingLosses=0 J
  QSL_Ideal_Switch : ee_lib/Semiconductors & Converters/MOSFET (Ideal, Switching)  port_option=ee.enum.controlport.ps  Rds=0.01 Ohm  Goff=1e-6 1/Ohm  Vth=2 V  diode_param=ee.enum.semiconductors.protectionDiode.nodynamics  diode_Vf=0.8 V  diode_Ron=0.001 Ohm  diode_Goff=1e-5 1/Ohm  diode_C=50e-9 F  diode_iRM=-235 A  diode_iF=300 A  diode_idot=-50 A/us  diode_trr_param=ee.enum.converters.diodeReverseParam.trr_factor  diode_trr_factor=3  diode_trr=15 us  diode_Qrr=1500 s*uA  ids_specify=off  ids_priority=None  ids=0 A  ids_nominal_specify=off  ids_nominal_value=1  ids_nominal_unit=A  vds_specify=off  vds_priority=None  vds=0 V  vds_nominal_specify=off  vds_nominal_value=1  vds_nominal_unit=V  vgs_specify=off  vgs_priority=None  vgs=0 V  vgs_nominal_specify=off  vgs_nominal_value=1  vgs_nominal_unit=V  thermal_loss_option=ee.enum.converters.thermalLossOption.constantvalues  Von_data=[0, 1.8, 3.2, 6, 10, 16; 0, 2, 5.5, 9.5, 15, 25] V  Tj=[298.15, 448.15] K  Iout_data=[0, 20, 40, 60, 80, 100] A  Eon_data=[0, 55.04, 124.57, 235.53, 362.12; 0, 71.25, 161.25, 304.88, 468.75] * 1e-6 J  Eoff_data=[0, 18, 30, 56.1, 76.5; 0, 22.5, 37.5, 70.13, 95.63] * 1e-6 J  Eon_data_3D=[zeros(2, 5, 3)] J  Eoff_data_3D=[zeros(2, 5, 3)] J  Tj_loss=[298.15, 448.15] K  Iout_data_loss=[0, 10, 20, 30, 40] A  tabulateWithVds=false  Vds_loss=[0, 150, 300] V  Eon_scalar=22.86e-3 J  Eoff_scalar=17.14e-3 J  Voff=300 V  Iout_scalar=600 A  useCurrentFromPreviousCycle=false  useVoltageFromPreviousCycle=false  diodeModelType=ee.enum.converters.diodeModelType.pwl  diodeTableType=ee.enum.diode.tableType.IfMat  diode_ReverseIVType=ee.enum.diode.diodeReverseIV.constant  diode_IfMat=[.07, .12, .19, 1.75, 4.24, 7.32, 11.2; .16, .3, .72, 2.14, 4.02, 6.35, 9.12] A  diode_VfMat=[.9, 1.15, 1.25, 1.5, 1.75, 2.17, 2.6, 2.85; .58, .68, .75, 1.1, 1.38, 1.77, 2.27, 2.7] V  diode_TjVec=[25, 125] degC  diode_VfVec=[.5, .7, .9, 1.3, 1.7, 2.1, 2.5] V  diode_IfVec=[.1, .2, .5, 1, 2, 4, 7, 10] A  diode_IrMat=[1e-06, 2e-06, 5e-06, 1e-05, 2.5e-05, 5e-05, .0001; 2e-06, 5e-06, 1e-05, 4e-05, 8e-05, .0002, .0005] A  diode_VrMat=[10, 100, 200, 250, 300, 325, 350; 10, 70, 160, 220, 270, 300, 320] V  diode_VrVec=[10, 20, 40, 50, 70, 80, 100] V  diode_IrVec=[1e-06, 2e-06, 5e-06, 1e-05, 2e-05, 5e-05, .0001] A  diode_Vr=-600 V  diode_Ls=150 nH  diode_Erec=0.03 J  diode_rec_loss_model=ee.enum.diode.reverseRecoveryModel.fixed  diode_ErecVal=0 J  diode_scaleWithIandV=true  diode_ErecMat=zeros(2, 3) J  diode_TjrecVec=[298.15, 398.15] K  diode_IfrecVec=[.1, 1, 10] A  diode_IrecVal=10 A  diode_VrecVal=10 V  diode_tFilter=1 / 1000 / 100 s  thermal_network_parameterization=ee.enum.thermalNetworkTopology.external  Rth=[.03, .2] K/W  Rth_Cauer=[.03, .1, .2] K/W  Rth_Foster=[.03, .2] K/W  thermal_mass_parameterization=ee.enum.thermalNetwork.timeconstant  thermal_mass=[3, 25] J/K  thermal_mass_Cauer=[3, 10, 25] J/K  thermal_mass_Foster=[33, 50] J/K  thermal_time_constant=[.1, 5] s  thermal_time_constant_Cauer=[.1, 1, 5] s  thermal_time_constant_Foster=[1, 10] s  thermal_mass_initial_temperatures=[25, 25] degC  thermal_mass_initial_temperatures_Cauer=[25, 25, 25] degC  junction_thermal_mass=0.1 J/K  Tvec_initial_Foster=[25, 25, 25, 25] degC  no_thermal_network=0  junction_temperature_specify=off  junction_temperature_priority=None  junction_temperature=25 degC  junction_temperature_nominal_specify=off  junction_temperature_nominal_value=1  junction_temperature_nominal_unit=degC  Qj_specify=off  Qj_priority=None  Qj=0 W  Qj_nominal_specify=off  Qj_nominal_value=1  Qj_nominal_unit=W  accumulatedSwitchingLosses_specify=off  accumulatedSwitchingLosses_priority=None  accumulatedSwitchingLosses=0 J
  Rds_QFH_50mOhm : fl_lib/Electrical/Electrical Elements/Resistor  R=0.05 Ohm  i_specify=off  i_priority=None  i=0 A  i_nominal_specify=off  i_nominal_value=1  i_nominal_unit=A  v_specify=off  v_priority=None  v=0 V  v_nominal_specify=off  v_nominal_value=1  v_nominal_unit=V
  Rds_QFL_50mOhm : fl_lib/Electrical/Electrical Elements/Resistor  R=0.05 Ohm  i_specify=off  i_priority=None  i=0 A  i_nominal_specify=off  i_nominal_value=1  i_nominal_unit=A  v_specify=off  v_priority=None  v=0 V  v_nominal_specify=off  v_nominal_value=1  v_nominal_unit=V
  Rds_QSH_50mOhm : fl_lib/Electrical/Electrical Elements/Resistor  R=0.05 Ohm  i_specify=off  i_priority=None  i=0 A  i_nominal_specify=off  i_nominal_value=1  i_nominal_unit=A  v_specify=off  v_priority=None  v=0 V  v_nominal_specify=off  v_nominal_value=1  v_nominal_unit=V
  Rds_QSL_50mOhm : fl_lib/Electrical/Electrical Elements/Resistor  R=0.05 Ohm  i_specify=off  i_priority=None  i=0 A  i_nominal_specify=off  i_nominal_value=1  i_nominal_unit=A  v_specify=off  v_priority=None  v=0 V  v_nominal_specify=off  v_nominal_value=1  v_nominal_unit=V
  AC_Line_In : PMIOPort  Side=Left
  AC_Neutral_In : PMIOPort  Port=2  Side=Left
  DC_Positive_Out : PMIOPort  Port=3  Side=Right
  DC_Negative_Out : PMIOPort  Port=4  Side=Right
  vin : Outport
  iin : Outport  Port=2
  vdc : Outport  Port=3
  wires:
  Gate_QFH/1 -> Gate_QFH_ToDouble/1
  Gate_QFH_ToDouble/1 -> Gate_QFH_0to10V/1
  Gate_QFH_0to10V/1 -> Gate_QFH_PS/1
  Gate_QFL/1 -> Gate_QFL_ToDouble/1
  Gate_QFL_ToDouble/1 -> Gate_QFL_0to10V/1
  Gate_QFL_0to10V/1 -> Gate_QFL_PS/1
  Gate_QSH/1 -> Gate_QSH_ToDouble/1
  Gate_QSH_ToDouble/1 -> Gate_QSH_0to10V/1
  Gate_QSH_0to10V/1 -> Gate_QSH_PS/1
  Gate_QSL/1 -> Gate_QSL_ToDouble/1
  Gate_QSL_ToDouble/1 -> Gate_QSL_0to10V/1
  Gate_QSL_0to10V/1 -> Gate_QSL_PS/1
  Input_Voltage_PS_to_SL/1 -> vin/1
  Input_Current_PS_to_SL/1 -> iin/1
  DC_Link_Voltage_PS_to_SL/1 -> vdc/1
  Gate_Precharge_Bypass/1 -> Precharge_Boolean_ToDouble/1
  Precharge_Boolean_ToDouble/1 -> Precharge_Command_0to10V/1
  Precharge_Command_0to10V/1 -> Precharge_Switch_PS/1
  Gate_Final_Precharge_Bypass/1 -> Final_Precharge_Boolean_ToDouble/1
  Final_Precharge_Boolean_ToDouble/1 -> Final_Precharge_Command_0to10V/1
  Final_Precharge_Command_0to10V/1 -> Final_Precharge_Switch_PS/1
  connections:
  Input_Voltage_Sensor/RConn2 -- Rds_QSH_50mOhm/RConn1 -- AC_Neutral_In/RConn1 -- Rds_QSL_50mOhm/RConn1
  Input_Current_Sensor/RConn2 -- Boost_Inductor_1mH_R80mOhm/LConn1
  QFL_Ideal_Switch/RConn1 -- Rds_QFL_50mOhm/LConn1
  QFL_Ideal_Switch/RConn2 -- QSL_Ideal_Switch/RConn2 -- DC_Negative_Out/RConn1 -- DC_Link_Voltage_Sensor/RConn2
  QSH_Ideal_Switch/RConn2 -- Rds_QSH_50mOhm/LConn1
  QSL_Ideal_Switch/RConn1 -- Rds_QSL_50mOhm/LConn1
  Gate_QFH_PS/RConn1 -- QFH_Ideal_Switch/LConn1
  Gate_QFL_PS/RConn1 -- QFL_Ideal_Switch/LConn1
  Gate_QSH_PS/RConn1 -- QSH_Ideal_Switch/LConn1
  Gate_QSL_PS/RConn1 -- QSL_Ideal_Switch/LConn1
  Input_Voltage_Sensor/RConn1 -- Input_Voltage_PS_to_SL/LConn1
  Input_Current_Sensor/RConn1 -- Input_Current_PS_to_SL/LConn1
  DC_Link_Voltage_Sensor/RConn1 -- DC_Link_Voltage_PS_to_SL/LConn1
  QSH_Ideal_Switch/RConn1 -- Rds_QFH_50mOhm/LConn1 -- DC_Positive_Out/RConn1 -- DC_Link_Voltage_Sensor/LConn1
  Boost_Inductor_1mH_R80mOhm/RConn1 -- Rds_QFL_50mOhm/RConn1 -- QFH_Ideal_Switch/RConn2
  Rds_QFH_50mOhm/RConn1 -- QFH_Ideal_Switch/RConn1
  Input_Voltage_Sensor/LConn1 -- Input_Precharge_Resistor_10Ohm/LConn1 -- AC_Line_In/RConn1 -- Input_Precharge_Bypass_Switch/LConn1
  Precharge_Switch_PS/RConn1 -- Input_Precharge_Bypass_Switch/RConn1
  Input_Precharge_Bypass_Switch/RConn2 -- Input_Precharge_Resistor_2Ohm/LConn1 -- Input_Precharge_Resistor_10Ohm/RConn1 -- Input_Final_Precharge_Bypass_Switch/LConn1
  Input_Current_Sensor/LConn1 -- Input_Precharge_Resistor_2Ohm/RConn1 -- Input_Final_Precharge_Bypass_Switch/RConn2
  Final_Precharge_Switch_PS/RConn1 -- Input_Final_Precharge_Bypass_Switch/RConn1
